simulink model "QPSKRx"  (R2017b)
settings: Solver=VariableStepDiscrete  StartTime=0.0  StopTime=inf  RelTol=1e-3
libraries: commdigbbndpm3 x3, commsdrhw_v2 x1
settings Model: Creator=Lab  LastModifiedBy=Lab

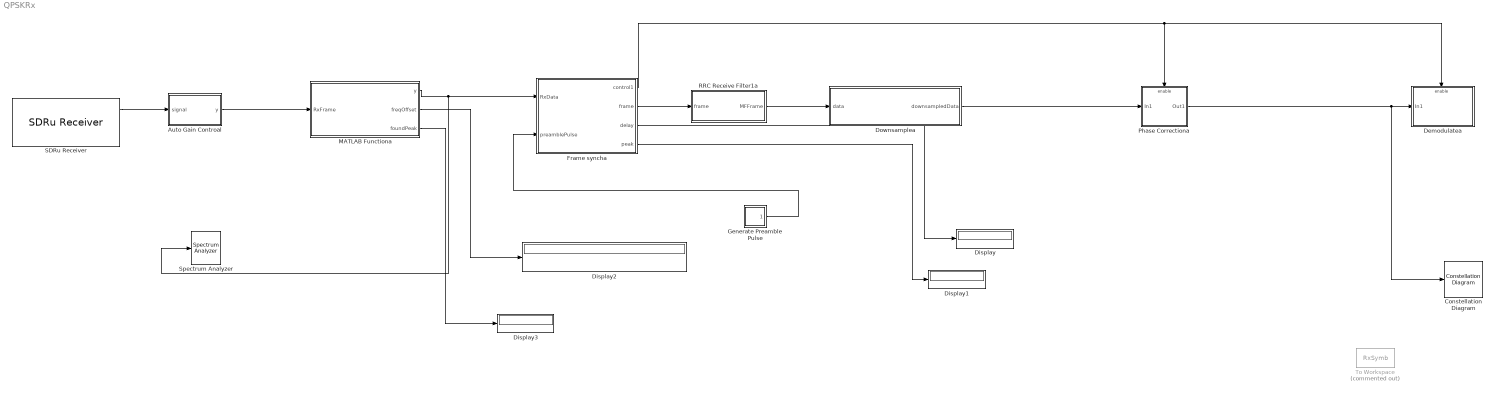
== system QPSKRx ==
  Auto Gain Controal : MATLAB Function  TreatAsAtomicUnit=on
  Constellation Diagram : ConstellationDiagram
  "Demodulatea " : Subsystem
  Display{,1..3} (4 alike) : Display
  Downsamplea : MATLAB Function  TreatAsAtomicUnit=on
  "Frame syncha " : MATLAB Function  TreatAsAtomicUnit=on
  "Generate Preamble Pulse " : Subsystem
  MATLAB Functiona : MATLAB Function  TreatAsAtomicUnit=on
  Phase Correctiona : Subsystem
  RRC Receive Filter1a : MATLAB Function  TreatAsAtomicUnit=on
  SDRu Receiver : commsdrhw_v2/SDRu Receiver  SourceLibraryInfo="This block requires <a href=\"http://www.mathworks.com/hardware-support/usrp.html\">Communications System Toolbox Support Package for USRP Radio</a>"  rxtx=rx  platform=N200/N210/USRP2  USRP2_IP='192.168.10.2'  USRP_IP_X300='192.168.10.2'  USRP_IP_X310='192.168.10.2'  USRP_serialNumB200=''  USRP_serialNumB210=''  ChannelMapping=1  centerFrequency=20e6  centerFrequencySrc=Dialog  loOffset=0  loOffsetSrc=Dialog  PPSSource=Internal  clockSource=Internal  masterClkRateB200=32e6  masterClkRateB210=32e6  masterClkRateX300=200e6  masterClkRateX310=200e6  masterClkRateParam=100e6  gain=31  gainSrc=Dialog  decimInterpSrc=Dialog  decimInterp=256  TransportDataType=int16  USRP2_IP_NUM=[49 57 50 46 49 54 56 46 49 48 46 50]  frameLength=(1696*3+1024*3)*2  outputDatatype=double  overrunUnderrunPort=off  sampleTime=1/390625  HOST_DATA_PORT=0  HOST_CONTROL_PORT=0  USRP2_DATA_PORT=0  USRP2_CONTROL_PORT=0  bufferMode=Guaranteed contiguous buffer  EnableBurstMode=on  NumFramesInBurst=2  USRP_ID='192.168.10.2'
      settings: SourceProductName=Communications System Toolbox Support Package for USRP(R) Radio  SourceProductBaseCode=USRP
  Spectrum Analyzer : SpectrumAnalyzer
  To Workspace : ToWorkspace  Commented=on  VariableName=RxSymb  SaveFormat=Structure  SampleTime=-1
      settings: Save2DSignal=2-D array (concatenate along first dimension)
  wires:
  MATLAB Functiona/2(freqOffset) -> Display2/1
  MATLAB Functiona/1(y) -> Spectrum Analyzer/1, "Frame syncha "/1(RxData)
  "Frame syncha "/4(peak) -> Display1/1
  "Frame syncha "/1(control1) -> "Demodulatea "/Enable, Phase Correctiona/Enable
  "Frame syncha "/3(delay) -> Display/1
  RRC Receive Filter1a/1(MFFrame) -> Downsamplea/1(data)
  "Frame syncha "/2(frame) -> RRC Receive Filter1a/1(frame)
  "Generate Preamble Pulse "/1(Out1) -> "Frame syncha "/2(preamblePulse)
  Phase Correctiona/1(Out1) -> Constellation Diagram/1, "Demodulatea "/1(In1)
  Downsamplea/1(downsampledData) -> Phase Correctiona/1(In1)
  SDRu Receiver/1 -> Auto Gain Controal/1(signal)
  Auto Gain Controal/1(y) -> MATLAB Functiona/1(RxFrame)
  MATLAB Functiona/3(foundPeak) -> Display3/1

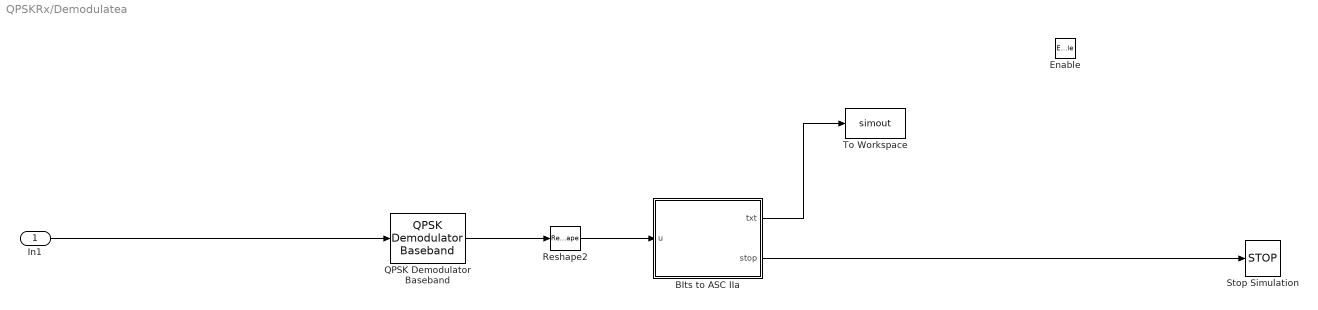
== system QPSKRx/Demodulatea  ==
  In1 : Inport
  Enable : EnablePort  StatesWhenEnabling=reset  PropagateVarSize=During execution
  BIts to ASC IIa : MATLAB Function  TreatAsAtomicUnit=on
  QPSK Demodulator Baseband : commdigbbndpm3/QPSK Demodulator Baseband  OutType=Bit  DecType=Hard decision  VarSource=Dialog  Variance=1  Dec=Gray  Ph=pi/4  outDtype1=Inherit via internal rule  outDtype2=Inherit via internal rule  derotateFactorWordLen=16  derotateFactorDataTypeStr=Inherit: Same word length as input  derotateFactorLastDataTypeStr=Inherit: Same word length as input
  Reshape2 : Reshape  OutputDimensionality=Row vector (2-D)
  Stop Simulation : Stop
  To Workspace : ToWorkspace  VariableName=simout  SaveFormat=Structure  SampleTime=-1
  wires:
  In1/1 -> QPSK Demodulator Baseband/1
  Reshape2/1 -> BIts to ASC IIa/1(u)
  QPSK Demodulator Baseband/1 -> Reshape2/1
  BIts to ASC IIa/1(txt) -> To Workspace/1
  BIts to ASC IIa/2(stop) -> Stop Simulation/1

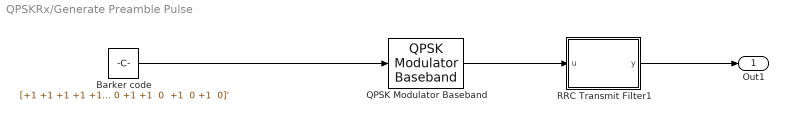
== system QPSKRx/Generate Preamble Pulse  ==
  Barker code : Constant  Value="[+1 +1 +1 +1 +1 0  0 +1 +1  0  +1  0 +1  0 +1 +1 +1 +1 +1 0  0 +1 +1  0  +1  0 +1  0]'"  VectorParams1D=off  SampleTime=-1
  QPSK Modulator Baseband : commdigbbndpm3/QPSK Modulator Baseband  InType=Bit  Enc=Gray  Ph=pi/4  outDtype=double  outWordLen=16  outUDDataType=sfix(16)  outFracLenMode=Best precision  outFracLen=15  outDataTypeStr=double  outLastDataTypeStr=double
  RRC Transmit Filter1 : MATLAB Function  TreatAsAtomicUnit=on
  Out1 : Outport
  wires:
  QPSK Modulator Baseband/1 -> RRC Transmit Filter1/1(u)
  Barker code/1 -> QPSK Modulator Baseband/1
  RRC Transmit Filter1/1(y) -> Out1/1

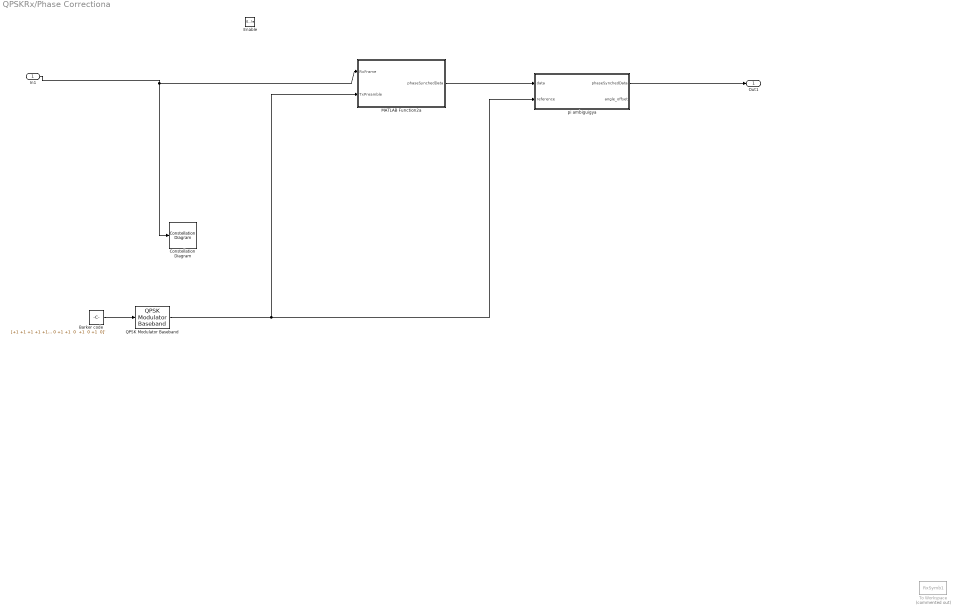
== system QPSKRx/Phase Correctiona ==
  In1 : Inport
  Enable : EnablePort  StatesWhenEnabling=reset  PropagateVarSize=During execution
  Barker code : Constant  Value="[+1 +1 +1 +1 +1 0  0 +1 +1  0  +1  0 +1  0 +1 +1 +1 +1 +1 0  0 +1 +1  0  +1  0 +1  0]'"  VectorParams1D=off  SampleTime=-1
  Constellation Diagram : ConstellationDiagram
  MATLAB Function2a : MATLAB Function  TreatAsAtomicUnit=on
  QPSK Modulator Baseband : commdigbbndpm3/QPSK Modulator Baseband  InType=Bit  Enc=Gray  Ph=pi/4  outDtype=double  outWordLen=16  outUDDataType=sfix(16)  outFracLenMode=Best precision  outFracLen=15  outDataTypeStr=double  outLastDataTypeStr=double
  To Workspace : ToWorkspace  Commented=on  VariableName=RxSymb1  SaveFormat=Structure  SampleTime=-1
      settings: Save2DSignal=2-D array (concatenate along first dimension)
  "pi ambiguigya " : MATLAB Function  TreatAsAtomicUnit=on
  Out1 : Outport
  wires:
  Barker code/1 -> QPSK Modulator Baseband/1
  QPSK Modulator Baseband/1 -> "pi ambiguigya "/2(reference), MATLAB Function2a/2(TxPreamble)
  In1/1 -> MATLAB Function2a/1(RxFrame), Constellation Diagram/1
  MATLAB Function2a/1(phaseSynchedData) -> "pi ambiguigya "/1(data)
  "pi ambiguigya "/1(phaseSynchedData) -> Out1/1

== matlab function QPSKRx/RRC Receive Filter1a ==
  data: MFFrame output size=[1656*3 1]; frame input size=[1696*3,1]
function MFFrame = fcn(frame)



rollOff = 0.6; 
span = 10; 
sps = 12; 

h = rcosdesign(rollOff, span, sps, 'sqrt'); 
MF = fliplr(conj(h));                             % Matched filter
y = conv(frame, MF); 


MFFrame = y(length(MF):end-length(MF)+1);         % Remove transients



end

== matlab function QPSKRx/MATLAB Functiona ==
  data: RxFrame input size=[(1696*3+1024*3)*2 1]; y output size=[(1696*3+1024*3)*2 1]; freqOffset output; foundPeak output
function [y,freqOffset, foundPeak] = freqCompensator(RxFrame)

    fs = (390625);                % Sample rate
    f_ref = 20e3;                   % Frequency of transmitted sinusoid
    NFFT = 2 ^ (nextpow2(fs));      % Number of NFFT-points
    
    frameLen = length(RxFrame); 
    
    
    

    
    
    buffer = complex(zeros(NFFT,1)); 
    buffer(end-frameLen+1:end) = RxFrame; 
    
    
    FFTFrame = abs(fft(buffer,NFFT)); 
    FFTFrameShift = fftshift(FFTFrame); 
    
    [~, idx] = max(FFTFrameShift); 
    offsetIdx = idx - NFFT/2; 
    
    
    deltaF = fs / NFFT; 
    foundPeak = deltaF * (offsetIdx-1);
    freqOffset = (f_ref - foundPeak); 
    
    
    
    
    t = (0:1/fs:(frameLen-1)/fs);
    
    
    y = RxFrame.*exp(1i*2*pi*freqOffset.*t'); 
    

end

== matlab function QPSKRx/Demodulatea /BIts to ASC IIa ==
  data: u input; txt output double size=[1 200]; stop output
function [txt, stop] = BITS2ASCII(u)


len=floor(length(u)/8);  
asc = ones(1,len);
multi=[128 64 32 16 8 4 2 1];


for i=1:len
 asc_bits=u(:, 8*i-7:8*i);
 ascnum = sum(asc_bits.*multi);
 asc(1,i)= ascnum;
end 
 
txt = asc; 
% Remove *-padding. 
% idx = find(asc==42);
% txt = zeros(1,idx(1)-1); 
% txt = asc(1:idx(1)-1); 

disp(char(txt))
stop = 1;       % Control signal to stop simulation 




end

== matlab function QPSKRx/Frame syncha  ==
  settings: updateMethod=DISCRETE
  data: control1 output; frame output size=[1696*3 1]; delay output; RxData input size=[(1696*3+1024*3)*2,1]; preamblePulse input; peak output
function [control1, frame,delay,peak]  = fcn(RxData, preamblePulse)

sps = 12;                 % Samples per symbol
frame_length = 414;      % Symbols per frame


% crosscorr = abs(xcorr(preamblePulse, RxData)); 
% [peak, idx] = max(crosscorr);

E_preamble = sum(abs(preamblePulse).^2); 
[corr, lag] = xcorr(RxData, preamblePulse); 
[peak, T] = max(abs(corr)); 
peak = peak/E_preamble; 
delay = lag(T);


if peak > 0.45 && delay < 2000*4 && delay > 500
    frame = RxData(delay+1:delay+frame_length*sps); 
    control1 = 1; 
else

    frame = zeros(frame_length*sps,1); 
    control1 = -1; 
end
%%
% len_pre=(1/2)*length(preamblePulse);
% window = ones(len_pre,1);
% CorrResult = RxData(1:end-len_pre).*conj(RxData(1+len_pre:end));
% corr_filted = real(conv(CorrResult,window))/len_pre;
% [peak2,index]=max(abs(corr_filted(1:end-sps*frame_length)));
% delay2= index - len_pre-delay;
% peak2=peak2/E_preamble;

== matlab function QPSKRx/Downsamplea ==
  settings: sampleTime=1/1.2e6
  data: data input; downsampledData output size=[414 1]
function downsampledData = fcn(data)


sps = 12 ; %downsample factor


downsampledData = downsample(data,sps); 


% downsampledData = complex(zeros(length(data)/sps, 1));
% tmp = complex(zeros(sps, length(data)/sps));
% 
% 
% tmp = reshape(data, [sps length(data)/sps]);
% downsampledData = conj(max((tmp)))';

end

== matlab function QPSKRx/Generate Preamble Pulse /RRC Transmit Filter1 ==
  data: u input; y output
function y = RRC(u)

rollOff = 0.6; 
span = 10; 
sps = 12; 

h = rcosdesign(rollOff, span, sps, 'sqrt'); 
symbs = upsample(u, sps); 
tmp = conv(symbs, h); 


y = tmp(1:end-length(h)+1);


end

== matlab function QPSKRx/Phase Correctiona/MATLAB Function2a ==
  data: RxFrame input size=[414 1]; phaseSynchedData output size=[414 1]; TxPreamble input
function phaseSynchedData = phaseSynch(RxFrame, TxPreamble)
N = length(RxFrame); 
phaseSynchedData = complex(zeros(N,1)); 



sps = 12; 
fs = ((100e6)/256)/sps; 
t = (0:1/fs:(N-1)/fs)'; 


N_pre = length(TxPreamble); 
t_pre = (0:1/fs:(N_pre-1)/fs)'; 


RxPreamble = RxFrame(1:14);

product = angle(TxPreamble.*conj(RxPreamble)); 

P = polyfit(t_pre, product, 1); 
freqOff = P(1)/(2*pi);
% freqOff = P(1);



data = RxFrame.*exp(1i*2*pi*freqOff.*t); 




% Correcting phase
a = 0;
mu = 1; 

for i = 1:length(data)
       ang = angle(data(i)) + a;            
       ang_correct = floor(ang*2/pi)*pi/2+pi/4; 
       e = ang_correct-ang; 
       a = a + mu*e;
       
       phaseSynchedData(i) = data(i) .* exp(1i*(a)); 

end








end

== matlab function QPSKRx/Auto Gain Controal ==
  data: signal input size=[(1696*3+1024*3)*2 1]; y output size=[(1696*3+1024*3)*2 1]
function y = AGC(signal)

%     signal = conj(signal); 
    N = length(signal);   % Length of signal
    upsample = 4*3; 
    Pout = 10*log10(1/upsample);   % Desired output in dB
    
    
    Pout_normal = 10.^(Pout/10); 
    E_normal = sum(abs(signal).^2); 
    
    coef = sqrt(Pout_normal*N/E_normal); 
    y = signal *coef; 
end

== matlab function QPSKRx/Phase Correctiona/pi ambiguigya  ==
  data: data input size=[414 1]; phaseSynchedData output size=[400 1]; reference input size=[14 1]; angle_offset output
function [phaseSynchedData, angle_offset] = fcn(data, reference)

preamble_data = data(1:14);
angle_offset = mean(wrapToPi(angle(reference)-angle(preamble_data)));


angle_offset = round(angle_offset*2/pi)*pi/2; 
phaseSynchedData = data .* exp(1i*(angle_offset)); 
phaseSynchedData = phaseSynchedData(15:end);
end



function lambda = wrapToPi(lambda)
%wrapToPi Wrap angle in radians to [-pi pi]
%
%   lambdaWrapped = wrapToPi(LAMBDA) wraps angles in LAMBDA, in radians,
%   to the interval [-pi pi] such that pi maps to pi and -pi maps to
%   -pi.  (In general, odd, positive multiples of pi map to pi and odd,
%   negative multiples of pi map to -pi.)
%
%   See also wrapTo2Pi, wrapTo180, wrapTo360.

% Copyright 2007-2008 The MathWorks, Inc.

q = (lambda < -pi) | (pi < lambda);
lambda(q) = wrapTo2Pi(lambda(q) + pi) - pi;
end



function lambda = wrapTo2Pi(lambda)
%wrapTo2Pi Wrap angle in radians to [0 2*pi]
%
%   lambdaWrapped = wrapTo2Pi(LAMBDA) wraps angles in LAMBDA, in radians,
%   to the interval [0 2*pi] such that zero maps to zero and 2*pi maps
%   to 2*pi. (In general, positive multiples of 2*pi map to 2*pi and
%   negative multiples of 2*pi map to zero.)
%
%   See also wrapToPi, wrapTo180, wrapTo360.

% Copyright 2007-2008 The MathWorks, Inc.

positiveInput = (lambda > 0);
lambda = mod(lambda, 2*pi);
lambda((lambda == 0) & positiveInput) = 2*pi;
end
